simulink model "SimpleTestFeeder_PQload"  (R2021b)
settings: Solver=ode4  StartTime=0.0  StopTime=20  FixedStep=50e-6  RelTol=1e-3  EnableMultiTasking=on
InitFcn:
  | Ts = 50e-6; %time step
undefined symbols (not defined in the file or in its folder): DiscIntNeverNeededParam, LoadLib, SinglePhase_PQLoad
libraries: spsSeriesRLCBranchLib x5, spsGroundLib x4, spsRMSLib x2, simulink x2, simulink_extras x2, spsDynamicLoadModel x2, spsVoltageMeasurementLib x2, spsCurrentMeasurementLib x1, spsPowerLib x1, spsACVoltageSourceLib x1, spsControlledCurrentSourceLib x1, spspowerguiLib x1
Description:
  | Model of a simple control system for use iin training.
settings Model: ARTEMISmethode_block_infos=$$__separator__$$  Creator=Paul Baracos  LastModifiedBy=gl8300
settings SolverCC: AlgebraicLoopSolver=TrustRegion
settings DataIOCC: LimitDataPoints=on  SaveFormat=Array  SignalLoggingSaveFormat=ModelDataLogs  SaveOutput=off  SaveTime=off  ReturnWorkspaceOutputs=off  SignalLoggingName=sigsOut
settings OptimizationCC: BlockReduction=off  BooleanDataType=off  OptimizeBlockIOStorage=off  BufferReuse=off  ExpressionFolding=off  LocalBlockOutputs=off  InitFltsAndDblsToZero=on  LifeSpan=inf
settings DebuggingCC: SaveWithParameterizedLinksMsg=none  UnderspecifiedInitializationDetection=Classic  MergeDetectMultiDrivingBlocksExec=none  SignalResolutionControl=TryResolveAllWithWarning  MultiTaskDSMMsg=warning  MultiTaskCondExecSysMsg=none  FcnCallInpInsideContextMsg=warning  SFUnexpectedBacktrackingDiag=warning  SFNoUnconditionalDefaultTransitionDiag=warning  SFExecutionAtInitializationDiag=none  SFMachineParentedDataDiag=warning  ArithmeticOperatorsInVariantConditions=warning
settings HardwareCC: ProdBitPerPointer=32  ProdBitPerSizeT=32  ProdBitPerPtrDiffT=32  ProdLargestAtomicFloat=None  ProdIntDivRoundTo=Undefined  ProdEndianess=Unspecified  ProdWordSize=32  ProdHWDeviceType=32-bit Generic  TargetBitPerPointer=64  TargetBitPerSizeT=64  TargetBitPerPtrDiffT=64  TargetLongLongMode=on  TargetIntDivRoundTo=Zero  TargetEndianess=LittleEndian  TargetWordSize=64  TargetHWDeviceType=MATLAB Host  ProdEqTarget=off
settings ModelReferenceCC: PropagateSignalLabelsOutOfModel=off
settings SFSimCC: SimUseLocalCustomCode=off  CustomCodeUndefinedFunction=UseInterfaceOnly
settings RTWCC: RTWUseLocalCustomCode=off
settings CodeAppCC: StateflowObjectComments=on
settings GRTTargetCC: TargetFcnLib=ansi_tfl_tmw.mat  TargetLangStandard=C89/C90 (ANSI)  CombineOutputUpdateFcns=off  GRTInterface=on
settings ConfigComp: CovMetricSettings=dw  CovSaveCumulativeToWorkspaceVar=on  CovSaveSingleToWorkspaceVar=on  CovExternalEMLEnable=off

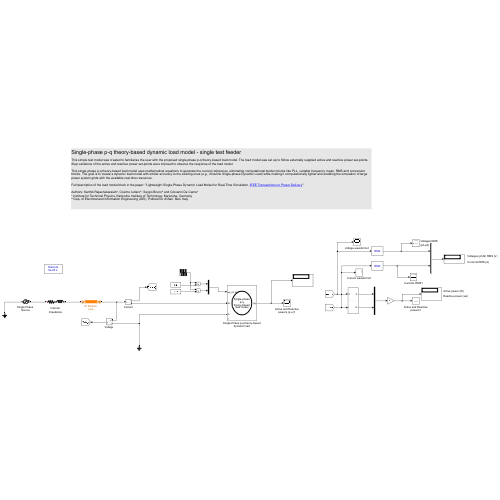
[thumbnail: Simulink's stored preview of the top-level diagram]
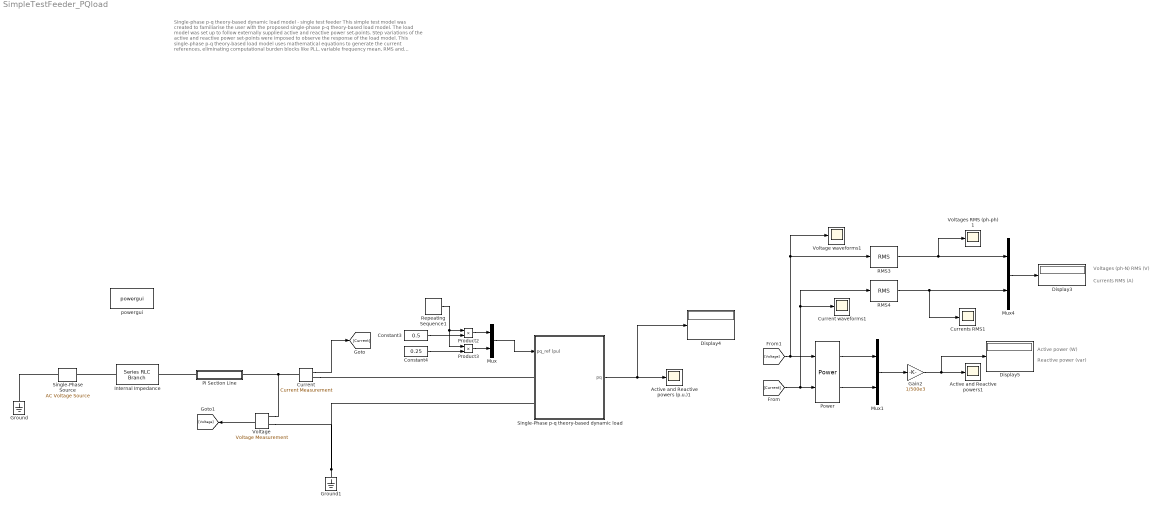
== system SimpleTestFeeder_PQload ==
  note: Single-phase p-q theory-based dynamic load model - single test feeder
      |
      | This simple test model was created to familiarise the user with the proposed single-phase p-q theory-based load model. The load model was set up to follow externally supplied active and reactive power set-points. Step variations of the active and reactive power set-points were imposed to observe the response of the load model.
      |
      | This single-phase p-q theory-based load model uses mathematical equations to generate the current references, eliminating computational burden blocks like PLL, variable frequency mean, RMS and conversion blocks. The goal is to create a dynamic load model with similar accuracy to the existing ones (e.g., Simulink Single-phase Dynamic Load) while making it computationally lighter and enabling the simulation of large power system grids with the available real-time resources.
      |
      | Full description of the load model block in the paper: "Lightweight Single-Phase Dynamic Load Model for Real-Time Simulation, IEEE Transactions on Power Delivery "
      |
      | Authors: Karthik Rajashekaraiah*, Cosimo Iurlaro^, Sergio Bruno^ and Giovanni De Carne*
      | * Institute for Technical Physics, Karlsruhe Institute of Technology, Karlsruhe, Germany
      | ^ Dep. of Electrical and Information Engineering (DEI), Politecnico di Bari, Bari, Italy
  note: Voltages (ph-N) RMS (V)
  note: Currents RMS (A)
  note: Active power (W)
  note: Reactive power (var)
  Active and Reactive powers (p.u.)1 : Scope
  Active and Reactive powers1 : Scope
  Constant3 : Constant  Value=0.5
  Constant4 : Constant  Value=0.25
  Current : spsCurrentMeasurementLib/Current Measurement  PhasorSimulation=off  OutputType=Complex  PSBequivalent=0
  Current waveforms1 : Scope
  Currents RMS1 : Scope
  Display3 : Display
  Display4 : Display
  Display5 : Display
  Gain2 : Gain  Gain=1/500e3
  Ground : spsGroundLib/Ground  LConnTagsString=a
  Ground1 : spsGroundLib/Ground  LConnTagsString=a
  Internal Impedance : spsSeriesRLCBranchLib/Series RLC Branch  LConnTagsString=__new0  RConnTagsString=__new0  BranchType=RL  Resistance=0.1e-9  Inductance=0.1e-9  SetiL0=off  InitialCurrent=0  Capacitance=1e-6  Setx0=off  InitialVoltage=0  Measurements=None
  Mux : Mux  Inputs=2
  Mux1 : Mux  Inputs=2
  Mux4 : Mux  Inputs=2
  PI Section Line : Subsystem  mask(Config302 (IEEE 34 Node Test Feeder)){fNom=60, length=1.6 * 1710 / 5280}
      mask prompts: fNom "Nominal frequency (Hz)"; length "Length (km)"
      mask Display:
      | patch([20 20 80 80], [30 70 70 30])
      | patch([0 0 20 20], [47 53 53 47])
      | patch([80 80 100 100], [47 53 53 47])
  Power : spsPowerLib/Power  Freq=60  Vinit=[1, 0]  Iinit=[1, 0]  Ts=0
      settings: SourceProductBaseCode=PS
  Product2 : Product
  Product3 : Product
  RMS3 : spsRMSLib/RMS  TrueRMS=on  Freq=50  RMSInit=0  Ts=0
  RMS4 : spsRMSLib/RMS  TrueRMS=on  Freq=50  RMSInit=0  Ts=0
  Repeating Sequence1 : simulink/Sources/Repeating Sequence  rep_seq_t=[0 5 5+Ts 10 10+Ts 15 15+Ts]  rep_seq_y=[1 1 1.1 1.1 0.9 0.9 1]
  Single-Phase Source : spsACVoltageSourceLib/AC Voltage Source  Amplitude=25e3*sqrt(2)/sqrt(3)  Phase=0  Frequency=60  SampleTime=0  Measurements=None  BusType=swing  Pref=10e3  Qref=0  Qmin=-inf  Qmax=+inf
  Single-Phase p-q theory-based dynamic load : Subsystem  AncestorBlock=LoadLib/SinglePhase_PQLoad  mask(Single-phase dynamic load){fnom=60, Vbase=25e3/sqrt(3), V0=1, S0=[4000 2000]/500e3, PQext=on, Kpi=[25 100*60], BasePower=500e3, n=[0 0], T=[0 0 0 0], Vmin=0.7, Freq_dep=on, FKpq=[0 0], Ts=50e-6}
      mask prompts: fnom "Nominal frequency [Hz]:"; Vbase "Nominal voltage [Vn(Vrms)]"; V0 "Initial positive-sequence voltage Vo [Mag(pu)]"; S0 "Active and reactive power at initial voltage [Po(pu) Qo(pu)]:"; PQext "External control of PQ"; Kpi "Active and Reactive power control parameters [Kp Ki]"; BasePower "Base Power (VA)"; n "[np, nq]:"; T "Time constants [Tp1 Tp2 Tq1 Tq2]  (s):"; Vmin "Minimum voltage Vmin (pu)"; Freq_dep "Frequency dependency"; FKpq "Frequency Dependency Gains [Kpf Kqf]"; Ts "Sample time (s)"
      mask help:
      | This single-phase p-q theory-based load model uses algebraic equations to generate the current references, eliminating computational burden blocks like PLL, mean, RMS, and conversion blocks. The goal is to create a dynamic load model with similar accuracy performance to the existing ones (e.g., Single-phase Dynamic Load) while making it computationally lighter and enabling the simulation of large power system grids with the available real-time resources.
      |
      | Full description of the load model block in the paper: "Lightweight Single-Phase Dynamic Load Model for Real-Time Simulation"
      |
      | Authors: K. Rajashekaraiah*, C. Iurlaro^, S. Bruno^ and G. De Carne*
      | * Institute for Technical Physics, Karlsruhe Institute of Technology, Karlsruhe, Germany
      | ^ Dep. of Electrical and Information Engineering (DEI), Politecnico di Bari, Bari, Italy
      |
      | Submitted and under review: IEEE Transactions on Power Delivery
      | Date of submission: 15/06/2024.
      | -----------
      | PKpi and QKpi contain the Kp and Ki gains of the PI controllers used to track the active and reactive power references, respectively. By modifying the values of these parameters, you can change the behaviour of the model to your liking.
      mask init:
      | wn=2*pi*fnom;
      | T1=1/wn;
      | Tp1=T(1);
      | Tp2=T(2);
      | Tq1=T(3);
      | Tq2=T(4);
      | P0=S0(1);
      | Q0=S0(2);
      | np=n(1);
      | nq=n(2);
      | Kpf=FKpq(1);
      | Kqf=FKpq(2);
      | K_SOGI = sqrt(2);
      | T=46;
      mask Callback PQext:
      | PQext = get_param(gcb,'PQext');
      | if strcmp(PQext,'on')
      |     set_param(gcb,'MaskEnables',{'on','on','off','off','on','on','on','off','off','off','off','off','on'});
      | else
      |     set_param(gcb,'MaskEnables',{'on','on','on','on','on','on','on','on','on','on','on','on','on'});
      | end
      mask Display:
      | %plot(-45,-45,45,45,[0,9,18,24,29,30,29,24,18,9,0,-9,-18,-24,-29,-30,-29,-24,-18,-9,0]*.9,[30,29,24,18,9,0,-9,-18,-24,-29,-30,-29,-24,-18,-9,0,9,18,24,29,30]*.9)
      | %plot([0,0,10,0,-10,0]*1.1,[15,-5,-5,-15,-5,-5]*1.1)
      | plot(-40,-40,40,40,[0,9,18,24,29,30,29,24,18,9,0,-9,-18,-24,-29,-30,-29,-24,-18,-9,0]*.9,[30,29,24,18,9,0,-9,-18,-24,-29,-30,-29,-24,-18,-9,0,9,18,24,29,30]*.9)
      | disp('Single-phase\np-q\ntheory-based\nload model')
  Voltage : spsVoltageMeasurementLib/Voltage Measurement  PhasorSimulation=off  OutputType=Complex  PSBequivalent=0
  Voltage waveforms1 : Scope
  Voltages RMS (ph-ph) 1 : Scope
  powergui : spspowerguiLib/powergui  Priority=1  SimulationMode=Discrete  SampleTime=Ts  frequency=Fn  Iterations=50  frequencyindice=0  Pbase=100e6  ErrMax=1e-4  UnitsV=kV  UnitsW=MW  buscounter=0  FunctionMessages=off  echomessages=off  EnableUseOfTLC=off  CurrentSourceSwitches=off  DisableSnubberDevices=off  DisableRonSwitches=off  DisableVfSwitches=off  DisplayEquations=off  AutomaticDiscreteSolvers=off  SolverType=Tustin/Backward Euler (TBE)  Interpol=off  ExternalGateDelay=off  methode=off  Ts=100  x0status=blocks  SPID=on  SwTol=0  HookPort=off  NonlinearTolerance=1e-4  nMaxIteration=100  ContinueOnMaxIteration=off  RestoreLinks=warning  ResistiveCurrentMeasurement=off  Frange=[0:2:500]  Ylog=off  Xlog=on  ShowGrid=off  save=off  variable=ZData  structure=0  ZoomFFT=off  StartTime=0.0  cycles=1  DisplayStyle=1  fundamental=60  FreqAxis=off  MaxFrequency=1000  frequencyindicesteady=1  RmsSteady=1  display=off
  wires:
  Single-Phase p-q theory-based dynamic load/1(pq) -> Display4/1, Active and Reactive powers (p.u.)1/1
  Current/1 -> [Current]
  Voltage/1 -> [Voltage]
  Repeating Sequence1/1 -> Product2/1, Product3/1
  Constant4/1 -> Product3/2
  Constant3/1 -> Product2/2
  Product2/1 -> Mux/1
  Mux/1 -> Single-Phase p-q theory-based dynamic load/1(pq_ref (pu))
  Product3/1 -> Mux/2
  Power/1 -> Mux1/1
  Power/2 -> Mux1/2
  Mux1/1 -> Gain2/1
  RMS4/1 -> Mux4/2, Currents RMS1/1
  RMS3/1 -> Voltages RMS (ph-ph) 1/1, Mux4/1
  [Current] -> RMS4/1, Current waveforms1/1, Power/2
  [Voltage] -> Power/1, Voltage waveforms1/1, RMS3/1
  Mux4/1 -> Display3/1
  Gain2/1 -> Display5/1, Active and Reactive powers1/1
  connections:
  Ground/LConn1 -- Single-Phase Source/LConn1
  Internal Impedance/LConn1 -- Single-Phase Source/RConn1
  PI Section Line/RConn1 -- Internal Impedance/RConn1
  Ground1/LConn1 -- Single-Phase p-q theory-based dynamic load/LConn2 -- Voltage/LConn2
  Current/RConn1 -- Single-Phase p-q theory-based dynamic load/LConn1
  Current/LConn1 -- Voltage/LConn1 -- PI Section Line/LConn1

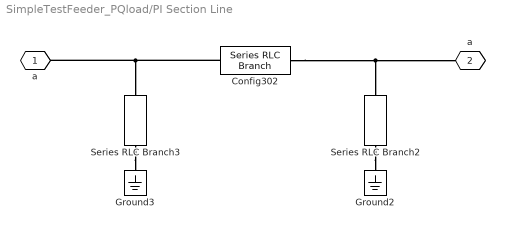
== system SimpleTestFeeder_PQload/PI Section Line ==
  Config302 : spsSeriesRLCBranchLib/Series RLC Branch  LConnTagsString=__new0  RConnTagsString=__new0  BranchType=RL  Resistance=2.7995 * length/1.6  Inductance=1.4855 / (2*fNom*pi) * length/1.6  SetiL0=off  InitialCurrent=0  Capacitance=1e-6  Setx0=off  InitialVoltage=0  Measurements=None
  Ground2 : spsGroundLib/Ground  LConnTagsString=a
  Ground3 : spsGroundLib/Ground  LConnTagsString=a
  Series RLC Branch2 : spsSeriesRLCBranchLib/Series RLC Branch  LConnTagsString=__new0  RConnTagsString=__new0  BranchType=C  Resistance=1  Inductance=1e-3  SetiL0=off  InitialCurrent=0  Capacitance=(4.2251*1e-6) / (2*fNom*pi) * length/1.6 / 2  Setx0=off  InitialVoltage=0  Measurements=None
  Series RLC Branch3 : spsSeriesRLCBranchLib/Series RLC Branch  LConnTagsString=__new0  RConnTagsString=__new0  BranchType=C  Resistance=1  Inductance=1e-3  SetiL0=off  InitialCurrent=0  Capacitance=(4.2251*1e-6) / (2*fNom*pi) * length/1.6 / 2  Setx0=off  InitialVoltage=0  Measurements=None
  a : PMIOPort  Tag=PMCPort  Side=Left
  "a " : PMIOPort  Tag=PMCPort  Port=2  Side=Right
  connections:
  Config302/LConn1 -- a/RConn1 -- Series RLC Branch3/LConn1
  Config302/RConn1 -- "a "/RConn1 -- Series RLC Branch2/LConn1
  Series RLC Branch2/RConn1 -- Ground2/LConn1
  Series RLC Branch3/RConn1 -- Ground3/LConn1

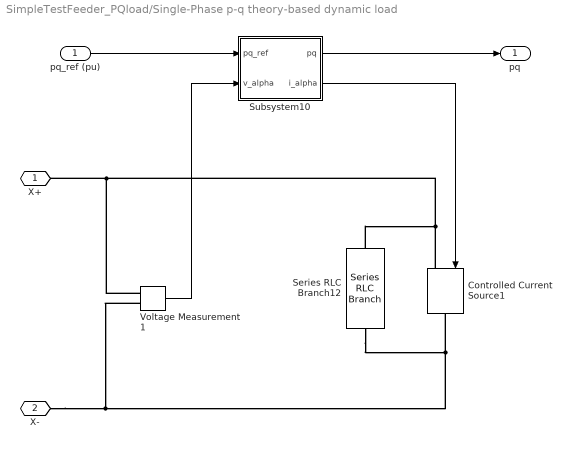
== system SimpleTestFeeder_PQload/Single-Phase p-q theory-based dynamic load ==
  pq_ref (pu) : Inport
  Controlled Current Source1 : spsControlledCurrentSourceLib/Controlled Current Source  Initialize=on  Source_Type=AC  Amplitude=0  Phase=0  Frequency=0  Measurements=None
  Series RLC Branch12 : spsSeriesRLCBranchLib/Series RLC Branch  LConnTagsString=__new0  RConnTagsString=__new0  BranchType=R  Resistance=1e8  Inductance=1e-3  SetiL0=off  InitialCurrent=0  Capacitance=1e-6  Setx0=off  InitialVoltage=0  Measurements=None
  Subsystem10 : Subsystem
  Voltage Measurement1 : spsVoltageMeasurementLib/Voltage Measurement  PhasorSimulation=off  OutputType=Complex  PSBequivalent=0
  X+ : PMIOPort  Side=Left
  X- : PMIOPort  Port=2  Side=Left
  pq : Outport
  wires:
  Subsystem10/1(pq) -> pq/1
  Subsystem10/2(i_alpha) -> Controlled Current Source1/1
  pq_ref (pu)/1 -> Subsystem10/1(pq_ref)
  Voltage Measurement1/1 -> Subsystem10/2(v_alpha)
  connections:
  X+/RConn1 -- Controlled Current Source1/LConn1 -- Series RLC Branch12/LConn1 -- Voltage Measurement1/LConn1
  Series RLC Branch12/RConn1 -- Controlled Current Source1/RConn1 -- X-/RConn1 -- Voltage Measurement1/LConn2

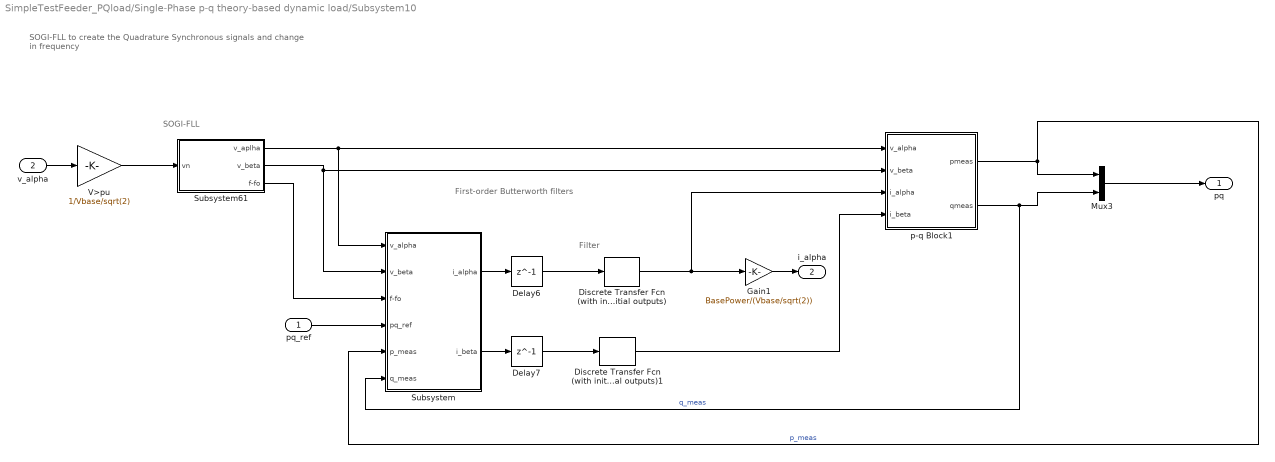
== system SimpleTestFeeder_PQload/Single-Phase p-q theory-based dynamic load/Subsystem10 ==
  note: SOGI-FLL to create the Quadrature Synchronous signals and change in frequency
  note: SOGI-FLL
  note: Filter
  note: First-order Butterworth filters
  pq_ref : Inport
  v_alpha : Inport  Port=2
  Delay6 : Delay  DelayLength=1  InitialCondition=0
  Delay7 : Delay  DelayLength=1  InitialCondition=0
  Discrete Transfer Fcn (with initial outputs) : simulink_extras/Additional Discrete/Discrete Transfer Fcn (with initial outputs)  N=[0.00933705475365587 0.00933705475365587]  D=[1 -0.981325890492688]  U0=0.01  Y0=0.01  TS=Ts
      settings: SourceProductBaseCode=SL
  Discrete Transfer Fcn (with initial outputs)1 : simulink_extras/Additional Discrete/Discrete Transfer Fcn (with initial outputs)  N=[0.00933705475365587 0.00933705475365587]  D=[1 -0.981325890492688]  U0=0.01  Y0=0.01  TS=Ts
      settings: SourceProductBaseCode=SL
  Gain1 : Gain  Gain=BasePower/(Vbase/sqrt(2))
  Mux3 : Mux  Inputs=2
  Subsystem : Subsystem
  Subsystem61 : Subsystem
  V>pu : Gain  Gain=1/Vbase/sqrt(2)
  p-q Block1 : MATLAB Function  TreatAsAtomicUnit=on
  pq : Outport
  i_alpha : Outport  Port=2
  wires:
  Subsystem61/1(v_aplha) -> Subsystem/1(v_alpha), p-q Block1/1(v_alpha)
  Discrete Transfer Fcn (with initial outputs)1/1 -> p-q Block1/4(i_beta)
  Discrete Transfer Fcn (with initial outputs)/1 -> p-q Block1/3(i_alpha), Gain1/1
  Gain1/1 -> i_alpha/1
  Delay7/1 -> Discrete Transfer Fcn (with initial outputs)1/1
  Delay6/1 -> Discrete Transfer Fcn (with initial outputs)/1
  Subsystem61/3(f-fo) -> Subsystem/3(f-fo)
  p-q Block1/1(pmeas) -> Mux3/1, Subsystem/5(p_meas)  "p_meas"
  v_alpha/1 -> V>pu/1
  pq_ref/1 -> Subsystem/4(pq_ref)
  Mux3/1 -> pq/1
  Subsystem/1(i_alpha) -> Delay6/1
  p-q Block1/2(qmeas) -> Mux3/2, Subsystem/6(q_meas)  "q_meas"
  Subsystem/2(i_beta) -> Delay7/1
  Subsystem61/2(v_beta) -> p-q Block1/2(v_beta), Subsystem/2(v_beta)
  V>pu/1 -> Subsystem61/1(vn)

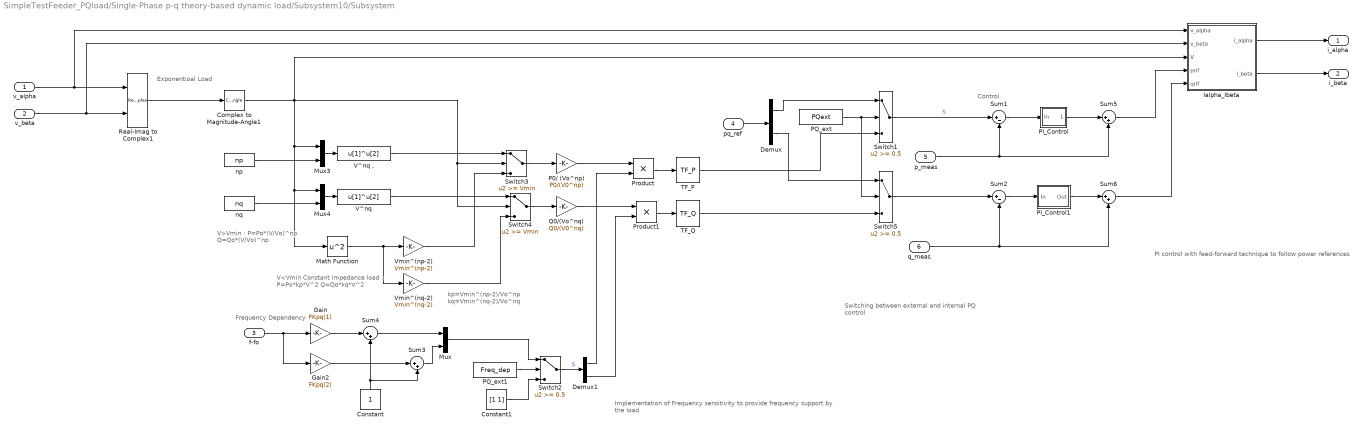
== system SimpleTestFeeder_PQload/Single-Phase p-q theory-based dynamic load/Subsystem10/Subsystem ==
  note: PI control with feed-forward
      | technique to follow power references
  note: Switching between external
      | and internal PQ control
  note: Implementation of Frequency sensitivity
      | to provide frequency support by the load
  note: Exponentioal Load
  note: Frequency Dependency
  note: Control
  note: V<Vmin
      | Constant impedance load :
      |  P=Po*kp*V^2
      | Q=Qo*kq*V^2
  note: kp=Vmin^(np-2)/Vo^np
      | kq=Vmin^(nq-2)/Vo^nq
  note: V>Vmin :
      |
      |    P=Po*(V/Vo)^np
      |    Q=Qo*(V/Vo)^np
  v_alpha : Inport
  v_beta : Inport  Port=2
  f-fo : Inport  Port=3
  pq_ref : Inport  Port=4
  p_meas : Inport  Port=5
  q_meas : Inport  Port=6
  Complex to Magnitude-Angle1 : ComplexToMagnitudeAngle  Output=Magnitude
  Constant : Constant
  Constant1 : Constant  Value=[1 1]
  Demux : Demux  Outputs=2
  Demux1 : Demux  Outputs=2
  Gain : Gain  Gain=FKpq(1)
  Gain2 : Gain  Gain=FKpq(2)
  Ialpha_Ibeta : Subsystem
  Math Function : Math  Operator=square  SignedPower=on  SaturateOnIntegerOverflow=on
  Mux : Mux  Inputs=2
  Mux3 : Mux  Inputs=2
  Mux4 : Mux  Inputs=2
  P0/ (Vo^np) : Gain  Gain=P0/(V0^np)  SaturateOnIntegerOverflow=on  OutDataTypeStr=Inherit: Same as input  ParamDataTypeStr=Inherit: Same as input
  PI_Control : Subsystem
  PI_Control1 : Subsystem
  PQ_ext : Constant  Value=PQext
  PQ_ext1 : Constant  Value=Freq_dep
  Product : Product
  Product1 : Product
  Q0/(Vo^nq) : Gain  Gain=Q0/(V0^nq)  SaturateOnIntegerOverflow=on  OutDataTypeStr=Inherit: Same as input  ParamDataTypeStr=Inherit: Same as input
  Real-Imag to Complex1 : RealImagToComplex
  Sum1 : Sum  Inputs=|+-
  Sum2 : Sum  Inputs=|+-
  Sum{3..6} (4 alike) : Sum  Inputs=|++
  Switch1 : Switch  Threshold=0.5  InputSameDT=on
  Switch2 : Switch  Threshold=0.5  InputSameDT=on
  Switch3 : Switch  Threshold=Vmin  InputSameDT=on
  Switch4 : Switch  Threshold=Vmin  InputSameDT=on
  Switch5 : Switch  Threshold=0.5  InputSameDT=on
  TF_P : spsDynamicLoadModel/Discrete/Positive Sequence  current/TF_P  T1=Tp1  T2=Tp2  V_Init=P0  Ts=Ts
      settings: SourceProductBaseCode=PS
  TF_Q : spsDynamicLoadModel/Discrete/Positive Sequence  current/TF_Q  T1=Tq1  T2=Tq2  V_Init=Q0  Ts=Ts
      settings: SourceProductBaseCode=PS
  V^nq : Fcn  Expr=u[1]^u[2]
  V^nq , : Fcn  Expr=u[1]^u[2]
  Vmin^(np-2) : Gain  Gain=Vmin^(np-2)  SaturateOnIntegerOverflow=on  OutDataTypeStr=Inherit: Same as input  ParamDataTypeStr=Inherit: Same as input
  Vmin^(nq-2) : Gain  Gain=Vmin^(nq-2)  SaturateOnIntegerOverflow=on  OutDataTypeStr=Inherit: Same as input  ParamDataTypeStr=Inherit: Same as input
  np : Constant  Value=np
  nq : Constant  Value=nq
  i_alpha : Outport
  i_beta : Outport  Port=2
  wires:
  Mux/1 -> Switch2/1
  Constant1/1 -> Switch2/3
  Complex to Magnitude-Angle1/1 -> Switch3/2, Switch4/2, Ialpha_Ibeta/3(V), Math Function/1, Mux4/1, Mux3/1
  Sum6/1 -> Ialpha_Ibeta/5(qrif)
  Sum5/1 -> Ialpha_Ibeta/4(prif)
  Product1/1 -> TF_Q/1
  Q0/(Vo^nq)/1 -> Product1/1
  Product/1 -> TF_P/1
  P0/ (Vo^np)/1 -> Product/1
  Demux1/2 -> Product1/2
  Gain2/1 -> Sum3/1
  Gain/1 -> Sum4/1
  Demux1/1 -> Product/2
  Sum4/1 -> Mux/1
  f-fo/1 -> Gain/1, Gain2/1
  PQ_ext1/1 -> Switch2/2
  Switch2/1 -> Demux1/1  "S"
  Sum3/1 -> Mux/2
  Constant/1 -> Sum4/2, Sum3/2
  Ialpha_Ibeta/1(i_alpha) -> i_alpha/1
  Ialpha_Ibeta/2(i_beta) -> i_beta/1
  Switch5/1 -> Sum2/1
  V^nq ,/1 -> Switch3/1
  TF_P/1 -> Switch1/3
  PQ_ext/1 -> Switch1/2, Switch5/2
  Mux3/1 -> V^nq ,/1
  Mux4/1 -> V^nq/1
  Math Function/1 -> Vmin^(nq-2)/1, Vmin^(np-2)/1
  Vmin^(np-2)/1 -> Switch3/3
  np/1 -> Mux3/2
  V^nq/1 -> Switch4/1
  v_alpha/1 -> Real-Imag to Complex1/1, Ialpha_Ibeta/1(v_alpha)
  Vmin^(nq-2)/1 -> Switch4/3
  Real-Imag to Complex1/1 -> Complex to Magnitude-Angle1/1
  Switch1/1 -> Sum1/1  "S"
  v_beta/1 -> Ialpha_Ibeta/2(v_beta), Real-Imag to Complex1/2
  Switch3/1 -> P0/ (Vo^np)/1
  nq/1 -> Mux4/2
  Switch4/1 -> Q0/(Vo^nq)/1
  Sum2/1 -> PI_Control1/1(In)
  Sum1/1 -> PI_Control/1(In)
  TF_Q/1 -> Switch5/3
  Demux/1 -> Switch1/1
  p_meas/1 -> Sum1/2, Sum5/2
  q_meas/1 -> Sum6/2, Sum2/2
  Demux/2 -> Switch5/1
  pq_ref/1 -> Demux/1
  PI_Control/1(Out) -> Sum5/1
  PI_Control1/1(Out) -> Sum6/1

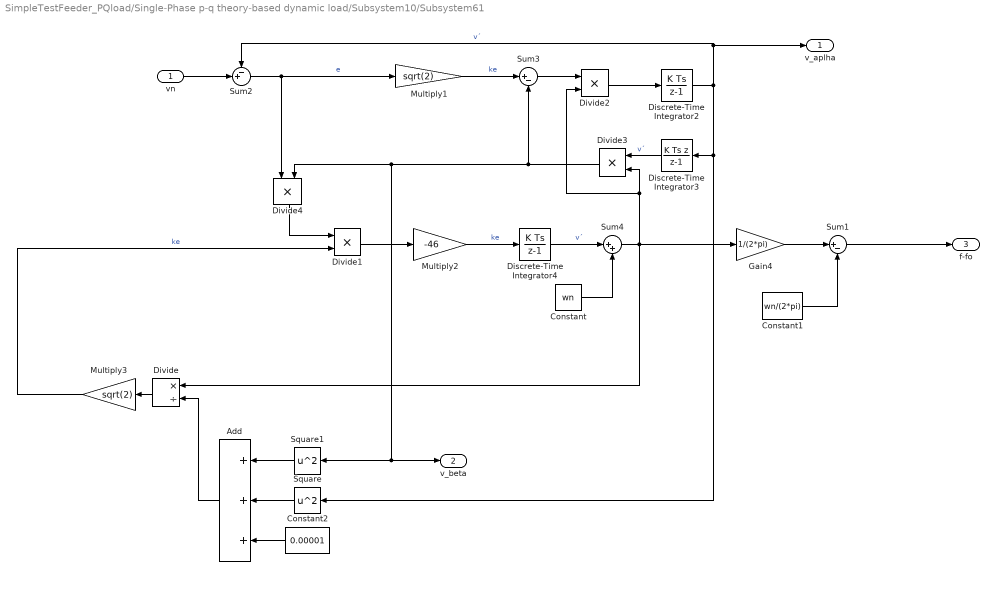
== system SimpleTestFeeder_PQload/Single-Phase p-q theory-based dynamic load/Subsystem10/Subsystem61 ==
  vn : Inport
  Add : Sum  Inputs=+++
  Constant : Constant  Value=wn
  Constant1 : Constant  Value=wn/(2*pi)
  Constant2 : Constant  Value=0.00001
  Discrete-Time Integrator2 : DiscreteIntegrator  SampleTime=-1  ICPrevOutput=DiscIntNeverNeededParam  ICPrevScaledInput=DiscIntNeverNeededParam
  Discrete-Time Integrator3 : DiscreteIntegrator  IntegratorMethod=Integration: Backward Euler  SampleTime=-1  ICPrevOutput=DiscIntNeverNeededParam  ICPrevScaledInput=DiscIntNeverNeededParam
  Discrete-Time Integrator4 : DiscreteIntegrator  SampleTime=-1  ICPrevOutput=DiscIntNeverNeededParam  ICPrevScaledInput=DiscIntNeverNeededParam
  Divide : Product  Inputs=*/
  Divide{1..4} (4 alike) : Product  Inputs=**
  Gain4 : Gain  Gain=1/(2*pi)
  Multiply1 : Gain  Gain=sqrt(2)
  Multiply2 : Gain  Gain=-46
  Multiply3 : Gain  Gain=sqrt(2)
  Square : Math  Operator=square  SaturateOnIntegerOverflow=on
  Square1 : Math  Operator=square  SaturateOnIntegerOverflow=on
  Sum1 : Sum  Inputs=|+-
  Sum2 : Sum  Inputs=-+|
  Sum3 : Sum  Inputs=|+-
  Sum4 : Sum  Inputs=|++
  v_aplha : Outport
  v_beta : Outport  Port=2
  f-fo : Outport  Port=3
  wires:
  Gain4/1 -> Sum1/1
  Sum4/1 -> Divide3/2, Divide2/2, Divide/1, Gain4/1
  Constant1/1 -> Sum1/2
  Sum1/1 -> f-fo/1
  Constant2/1 -> Add/3
  Multiply3/1 -> Divide1/2  "ke"
  Divide4/1 -> Divide1/1
  Divide1/1 -> Multiply2/1
  Divide/1 -> Multiply3/1
  Add/1 -> Divide/2
  Square/1 -> Add/2
  Square1/1 -> Add/1
  Sum3/1 -> Divide2/1
  Multiply1/1 -> Sum3/1  "ke"
  Multiply2/1 -> Discrete-Time Integrator4/1  "ke"
  Constant/1 -> Sum4/2
  Discrete-Time Integrator3/1 -> Divide3/1  "v´"
  Sum2/1 -> Multiply1/1, Divide4/1  "e"
  Discrete-Time Integrator4/1 -> Sum4/1  "v´"
  Discrete-Time Integrator2/1 -> Sum2/1, v_aplha/1, Discrete-Time Integrator3/1, Square/1  "v´"
  Divide2/1 -> Discrete-Time Integrator2/1
  vn/1 -> Sum2/2
  Divide3/1 -> Sum3/2, v_beta/1, Square1/1, Divide4/2

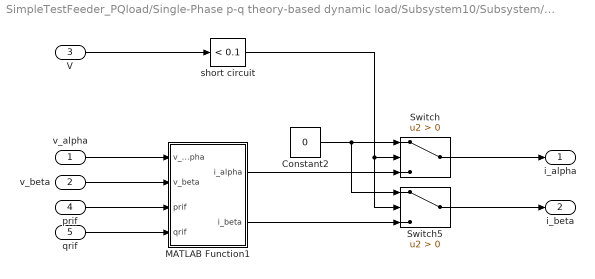
== system SimpleTestFeeder_PQload/Single-Phase p-q theory-based dynamic load/Subsystem10/Subsystem/Ialpha_Ibeta ==
  v_alpha : Inport
  v_beta : Inport  Port=2
  V : Inport  Port=3
  prif : Inport  Port=4
  qrif : Inport  Port=5
  Constant2 : Constant  Value=0
  MATLAB Function1 : MATLAB Function  TreatAsAtomicUnit=on
  Switch : Switch  Criteria=u2 > Threshold
  Switch5 : Switch  Criteria=u2 > Threshold
  short circuit : simulink/Logic and Bit Operations/Compare To Constant  relop=<  const=0.1  OutDataTypeStr=boolean
  i_alpha : Outport
  i_beta : Outport  Port=2
  wires:
  short circuit/1 -> Switch/2, Switch5/2
  Switch5/1 -> i_beta/1
  Switch/1 -> i_alpha/1
  v_beta/1 -> MATLAB Function1/2(v_beta)
  prif/1 -> MATLAB Function1/3(prif)
  MATLAB Function1/1(i_alpha) -> Switch/3
  Constant2/1 -> Switch5/1, Switch/1
  qrif/1 -> MATLAB Function1/4(qrif)
  v_alpha/1 -> MATLAB Function1/1(v_alpha)
  V/1 -> short circuit/1
  MATLAB Function1/2(i_beta) -> Switch5/3

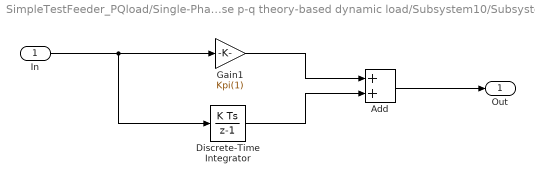
== system SimpleTestFeeder_PQload/Single-Phase p-q theory-based dynamic load/Subsystem10/Subsystem/PI_Control ==
  In : Inport
  Add : Sum
  Discrete-Time Integrator : DiscreteIntegrator  gainval=Kpi(2)  SampleTime=-1  ICPrevOutput=DiscIntNeverNeededParam  ICPrevScaledInput=DiscIntNeverNeededParam
  Gain1 : Gain  Gain=Kpi(1)
  Out : Outport
  wires:
  Discrete-Time Integrator/1 -> Add/2
  Add/1 -> Out/1
  Gain1/1 -> Add/1
  In/1 -> Gain1/1, Discrete-Time Integrator/1

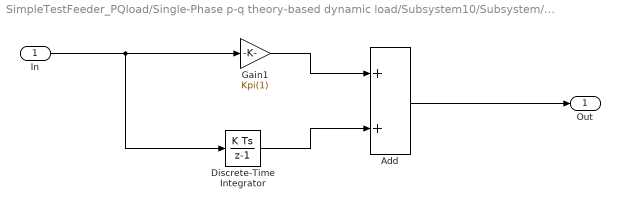
== system SimpleTestFeeder_PQload/Single-Phase p-q theory-based dynamic load/Subsystem10/Subsystem/PI_Control1 ==
  In : Inport
  Add : Sum
  Discrete-Time Integrator : DiscreteIntegrator  gainval=Kpi(2)  SampleTime=-1  ICPrevOutput=DiscIntNeverNeededParam  ICPrevScaledInput=DiscIntNeverNeededParam
  Gain1 : Gain  Gain=Kpi(1)
  Out : Outport
  wires:
  Add/1 -> Out/1
  Discrete-Time Integrator/1 -> Add/2
  Gain1/1 -> Add/1
  In/1 -> Gain1/1, Discrete-Time Integrator/1

== matlab function SimpleTestFeeder_PQload/Single-Phase p-q theory-based dynamic load/Subsystem10/Subsystem/Ialpha_Ibeta/MATLAB Function1 ==
  data: v_alpha input; i_alpha output; v_beta input; prif input; qrif input; i_beta output

function [i_alpha,i_beta]= fcn(v_alpha,v_beta,prif,qrif)
i_alpha=(v_alpha.*prif+v_beta.*qrif)/(v_alpha.^2+v_beta.^2);
i_beta=(v_beta.*prif-v_alpha.*qrif)/(v_alpha.^2+v_beta.^2);

== matlab function SimpleTestFeeder_PQload/Single-Phase p-q theory-based dynamic load/Subsystem10/p-q Block1 ==
  data: v_alpha input; pmeas output; v_beta input; i_alpha input; i_beta input; qmeas output
function [pmeas,qmeas]= fcn(v_alpha,v_beta,i_alpha,i_beta)

pmeas=v_alpha.*i_alpha+v_beta.*i_beta;
qmeas=v_beta.*i_alpha-v_alpha.*i_beta;
